simulink model "MSIP_Speed_Control_abc1a_2025a_no_VSC_no_Bspline"  (R2025a)
settings: Solver=FixedStepAuto  StartTime=0.0  StopTime=150  FixedStep=1e-4  MaxStep=1e-3  RelTol=1e-3
model workspace (MAT data in the model file):
  Freq = 60
values from neighbouring files (symbols this model uses):
  alpha0_wMS = (b_MS*Rs_MS/(J_MS*Lq_MS)) +               (3*np_MS*np_MS*lambda_MS*lambda_MS/              (2*J_MS*Lq_MS))    (= 296.519413831)    [data_MSIP_julio2025.m]
  alpha1_wMS = (Rs_MS/Lq_MS) + (b_MS/J_MS)    (= 7.15599341383)    [data_MSIP_julio2025.m]
  b_MS = 1e-3    (= 0.001)    [data_MSIP_julio2025.m]
  beta0_wMS = Pw^2    (= 400)    [data_MSIP_julio2025.m]
  beta1_wMS = 2*Pw    (= 40)    [data_MSIP_julio2025.m]
  beta_d_MS = pd_MS    (= 40)    [data_MSIP_julio2025.m]
  gamq = 2*J_MS*Lq_MS/(3*np_MS*lambda_MS)    (= 0.00452625826005)    [data_MSIP_julio2025.m]
  J_MS = 1e-1    (= 0.1)    [data_MSIP_julio2025.m]
  lambda_MS = 67.09e-2    (= 0.6709)    [data_MSIP_julio2025.m]
  Ld_MS = 22.1e-3    (= 0.0221)    [data_MSIP_julio2025.m]
  Lq_MS = 91.1e-3    (= 0.0911)    [data_MSIP_julio2025.m]
  np_MS = 2    [data_MSIP_julio2025.m]
  Rs_MS = 6.51e-1    (= 0.651)    [data_MSIP_julio2025.m]
undefined symbols (not defined in the file or in its folder): plecs
libraries: plecslib_extras2 x2, spsRMSLib x2
settings Model: SimulationMode=accelerator  PauseTimes=0.01  Creator=RUBEN TAPIA OLVERA  LastModifiedBy=avalder
settings SolverCC: AlgebraicLoopSolver=TrustRegion
settings DataIOCC: ReturnWorkspaceOutputs=off
settings OptimizationCC: LifeSpan=inf
settings DebuggingCC: MaxConsecutiveZCsMsg=none  UnconnectedInputMsg=warning  UnconnectedOutputMsg=warning  UnconnectedLineMsg=warning  SFUnexpectedBacktrackingDiag=warning  SFNoUnconditionalDefaultTransitionDiag=warning  SFExecutionAtInitializationDiag=none  ArithmeticOperatorsInVariantConditions=warning
settings ModelReferenceCC: EnableRefExpFcnMdlSchedulingChecks=on
settings SFSimCC: SimUseLocalCustomCode=off  CustomCodeUndefinedFunction=UseInterfaceOnly
settings RTWCC: RTWUseLocalCustomCode=off  GPUComputeCapability=3.5
settings CodeAppCC: StateflowObjectComments=on
settings GRTTargetCC: TargetLangStandard=C89/C90 (ANSI)
settings ConfigComp: CovMetricSettings=dw  CovSaveCumulativeToWorkspaceVar=on  CovSaveSingleToWorkspaceVar=on  CovExternalEMLEnable=off
settings SimscapeCC: SimscapeNormalizeSystem=off

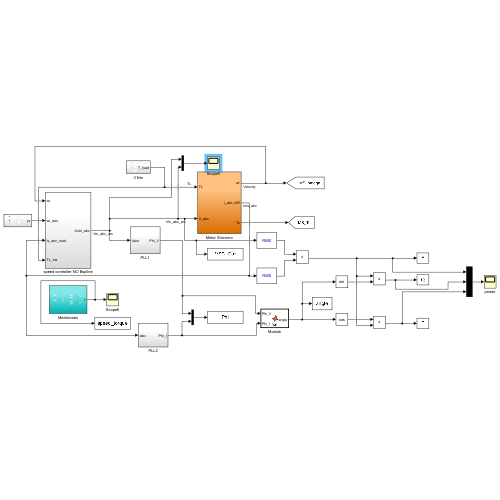
[thumbnail: Simulink's stored preview of the top-level diagram]
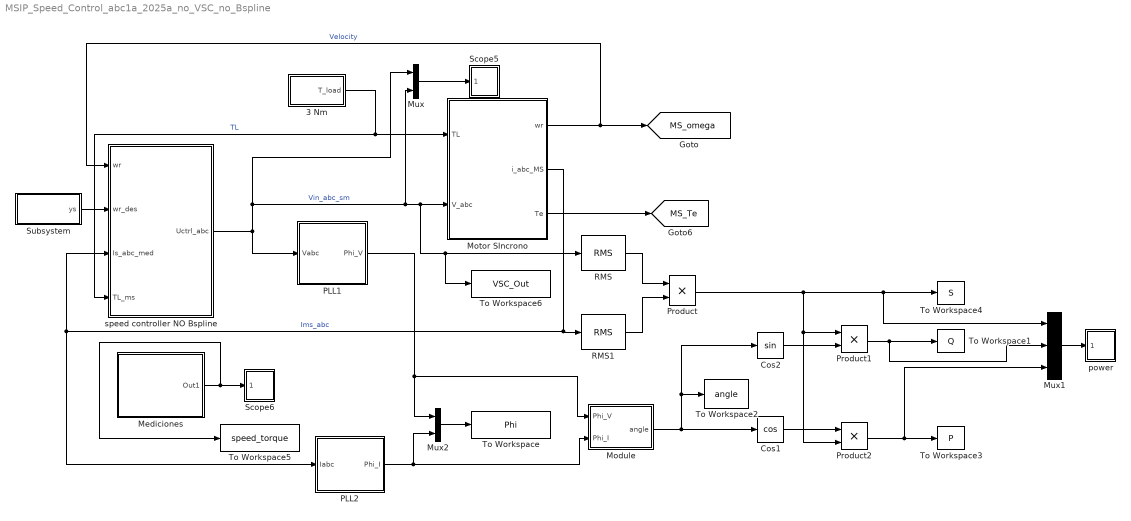
== system MSIP_Speed_Control_abc1a_2025a_no_VSC_no_Bspline ==
  3 Nm : Subsystem
  Cos1 : Trigonometry  Operator=cos
  Cos2 : Trigonometry
  Mediciones : Subsystem
  Module : MATLAB Function  TreatAsAtomicUnit=on
  Motor SIncrono : Subsystem
  Mux : Mux  Inputs=2
  Mux1 : Mux  Inputs=3
  Mux2 : Mux  Inputs=2
  PLL1 : Subsystem
  PLL2 : Subsystem
  Product : Product
  Product1 : Product
  Product2 : Product
  RMS : spsRMSLib/RMS  TrueRMS=on  Freq=Freq  RMSInit=0  Ts=0
  RMS1 : spsRMSLib/RMS  TrueRMS=on  Freq=Freq  RMSInit=0  Ts=0
  Scope5 : Subsystem  LoadFcn=plecs('sl', 300);  InitFcn=plecs('sl', 314);  StartFcn=plecs('sl', 308);  StopFcn=plecs('sl', 309);  mask{Settings=<binary blob, 776 chars, not shown>}
      mask init:
      | plecs('sl', 315);
      settings: CopyFcn=plecs('sl', 303);  DeleteFcn=plecs('sl', 305);  UndoDeleteFcn=plecs('sl', 306);  PreSaveFcn=plecs('sl', 311);  NameChangeFcn=plecs('sl', 310);  DestroyFcn=plecs('sl', 307);  OpenFcn=plecs('sl', 302);  ErrorFcn=plerrorfcn
      mask Display: plot([0.1 0.9 0.9 0.1 0.1], [0.9 0.9 0.5 0.5 0.9])
  Scope6 : Subsystem  LoadFcn=plecs('sl', 300);  InitFcn=plecs('sl', 314);  StartFcn=plecs('sl', 308);  StopFcn=plecs('sl', 309);  mask{Settings=<binary blob, 752 chars, not shown>}
      mask init:
      | plecs('sl', 315);
      settings: CopyFcn=plecs('sl', 303);  DeleteFcn=plecs('sl', 305);  UndoDeleteFcn=plecs('sl', 306);  PreSaveFcn=plecs('sl', 311);  NameChangeFcn=plecs('sl', 310);  DestroyFcn=plecs('sl', 307);  OpenFcn=plecs('sl', 302);  ErrorFcn=plerrorfcn
      mask Display: plot([0.1 0.9 0.9 0.1 0.1], [0.9 0.9 0.5 0.5 0.9])
  Subsystem : Subsystem
  To Workspace : ToWorkspace  VariableName=Phi  SaveFormat=Timeseries  SampleTime=-1
  To Workspace1 : ToWorkspace  VariableName=Q  SaveFormat=Timeseries  SampleTime=-1
  To Workspace2 : ToWorkspace  VariableName=angle  SaveFormat=Timeseries  SampleTime=-1
  To Workspace3 : ToWorkspace  VariableName=P  SaveFormat=Timeseries  SampleTime=-1
  To Workspace4 : ToWorkspace  VariableName=S  SaveFormat=Timeseries  SampleTime=-1
  To Workspace5 : ToWorkspace  VariableName=speed_torque  SaveFormat=Timeseries  SampleTime=-1
  To Workspace6 : ToWorkspace  VariableName=VSC_Out  SaveFormat=Timeseries  SampleTime=-1
  power : Subsystem  LoadFcn=plecs('sl', 300);  InitFcn=plecs('sl', 314);  StartFcn=plecs('sl', 308);  StopFcn=plecs('sl', 309);  mask{Settings=<binary blob, 756 chars, not shown>}
      mask init:
      | plecs('sl', 315);
      settings: CopyFcn=plecs('sl', 303);  DeleteFcn=plecs('sl', 305);  UndoDeleteFcn=plecs('sl', 306);  PreSaveFcn=plecs('sl', 311);  NameChangeFcn=plecs('sl', 310);  DestroyFcn=plecs('sl', 307);  OpenFcn=plecs('sl', 302);  ErrorFcn=plerrorfcn
      mask Display: plot([0.1 0.9 0.9 0.1 0.1], [0.9 0.9 0.5 0.5 0.9])
  speed controller NO Bspline : Subsystem
  tag scope: MS_Te=global, MS_omega=global
  wires:
  Motor SIncrono/1(wr) -> speed controller NO Bspline/1(wr), [MS_omega]  "Velocity"
  3 Nm/1(T_load) -> speed controller NO Bspline/4(TL_ms), Motor SIncrono/1(TL)  "TL"
  Motor SIncrono/3(Te) -> [MS_Te]
  Motor SIncrono/2(i_abc_MS) -> RMS1/1, speed controller NO Bspline/3(Is_abc_med), PLL2/1(Iabc)  "Ims_abc"
  Subsystem/1(ys) -> speed controller NO Bspline/2(wr_des)
  Mux2/1 -> To Workspace/1
  Module/1(angle) -> Cos1/1, To Workspace2/1, Cos2/1
  PLL1/1(Phi_V) -> Mux2/1, Module/1(Phi_V)
  PLL2/1(Phi_I) -> Module/2(Phi_I), Mux2/2
  speed controller NO Bspline/1(Uctrl_abc) -> Mux/2, Motor SIncrono/2(V_abc), To Workspace6/1, RMS/1, Mux/1, PLL1/1(Vabc)  "Vin_abc_sm"
  Product/1 -> Product2/2, Product1/1, Mux1/1, To Workspace4/1
  RMS/1 -> Product/1
  RMS1/1 -> Product/2
  Mux/1 -> Scope5/1(1)
  Mediciones/1(Out1) -> To Workspace5/1, Scope6/1(1)
  Cos2/1 -> Product1/2
  Cos1/1 -> Product2/1
  Product1/1 -> Mux1/2, To Workspace1/1
  Product2/1 -> Mux1/3, To Workspace3/1
  Mux1/1 -> power/1(1)

== system MSIP_Speed_Control_abc1a_2025a_no_VSC_no_Bspline/3 Nm ==
  Add : Sum  Inputs=+++
  TL1 : MATLAB Function  TreatAsAtomicUnit=on
  TL2 : MATLAB Function  TreatAsAtomicUnit=on
  TL3 : MATLAB Function  TreatAsAtomicUnit=on
  Tiempo1 : Clock
  T_load : Outport
  tag scope: TL_MS=global
  wires:
  Tiempo1/1 -> TL3/1(t), TL2/1(t), TL1/1(t)
  TL3/1(T_load3) -> Add/3
  TL1/1(T_load) -> Add/1
  TL2/1(T_load2) -> Add/2
  Add/1 -> T_load/1, [TL_MS]

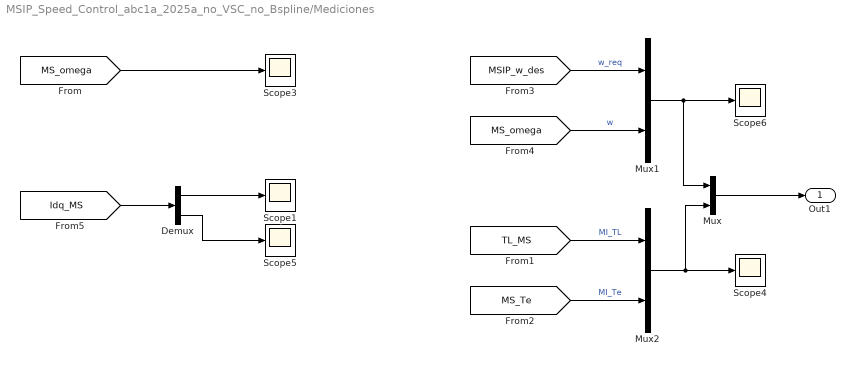
== system MSIP_Speed_Control_abc1a_2025a_no_VSC_no_Bspline/Mediciones ==
  Demux : Demux  Outputs=2
  Mux : Mux  Inputs=2
  Mux1 : Mux  Inputs=2
  Mux2 : Mux  Inputs=2
  Scope{1,3..6} (5 alike) : Scope
      Scope1 settings: Title=Currents  ActiveDisplayYMinimum=-0.00105  ActiveDisplayYMaximum=0.01123  DataLoggingVariableName=ScopeData3
      Scope3 settings: ActiveDisplayYMinimum=-1  ActiveDisplayYMaximum=1
      Scope4 settings: ActiveDisplayYMinimum=-1  ActiveDisplayYMaximum=1  DataLoggingVariableName=ScopeData4
      Scope5 settings: Title=Currents  ActiveDisplayYMinimum=-0.003  ActiveDisplayYMaximum=0.00033
      Scope6 settings: ActiveDisplayYMinimum=-23.57031  ActiveDisplayYMaximum=212.1328
  Out1 : Outport
  wires:
  [MS_omega] -> Scope3/1
  [TL_MS] -> Mux2/1  "MI_TL"
  Mux2/1 -> Mux/2, Scope4/1
  [MS_Te] -> Mux2/2  "MI_Te"
  [Idq_MS] -> Demux/1
  Demux/1 -> Scope1/1
  Demux/2 -> Scope5/1
  [MS_omega] -> Mux1/2  "w"
  [MSIP_w_des] -> Mux1/1  "w_req"
  Mux1/1 -> Mux/1, Scope6/1
  Mux/1 -> Out1/1

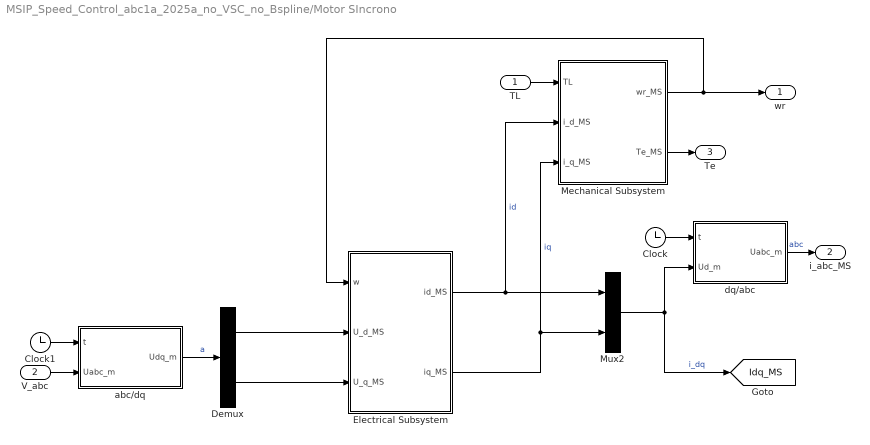
== system MSIP_Speed_Control_abc1a_2025a_no_VSC_no_Bspline/Motor SIncrono ==
  TL : Inport
  V_abc : Inport  Port=2
  Clock : Clock
  Clock1 : Clock
  Demux : Demux  Outputs=2
  Electrical Subsystem : Subsystem
  Mechanical Subsystem : Subsystem
  Mux2 : Mux  Inputs=2
  abc/dq : Subsystem
  dq/abc : Subsystem
  wr : Outport
  i_abc_MS : Outport  Port=2
  Te : Outport  Port=3
  tag scope: Idq_MS=global
  wires:
  Mechanical Subsystem/1(wr_MS) -> wr/1, Electrical Subsystem/1(w)
  TL/1 -> Mechanical Subsystem/1(TL)
  Mechanical Subsystem/2(Te_MS) -> Te/1
  Demux/1 -> Electrical Subsystem/2(U_d_MS)
  Demux/2 -> Electrical Subsystem/3(U_q_MS)
  Electrical Subsystem/1(id_MS) -> Mux2/1, Mechanical Subsystem/2(i_d_MS)  "id"
  Electrical Subsystem/2(iq_MS) -> Mechanical Subsystem/3(i_q_MS), Mux2/2  "iq"
  Mux2/1 -> dq/abc/2(Ud_m), [Idq_MS]  "i_dq"
  Clock/1 -> dq/abc/1(t)
  dq/abc/1(Uabc_m) -> i_abc_MS/1  "abc"
  Clock1/1 -> abc/dq/1(t)
  abc/dq/1(Udq_m) -> Demux/1  "a"
  V_abc/1 -> abc/dq/2(Uabc_m)

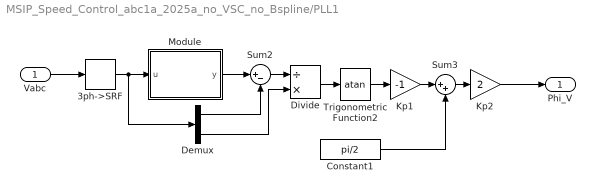
== system MSIP_Speed_Control_abc1a_2025a_no_VSC_no_Bspline/PLL1 ==
  Vabc : Inport
  3ph->SRF : plecslib_extras2/Transformations/3ph->SRF
      settings: SourceProductName=PLECS Extras
  Constant1 : Constant  Value=pi/2
  Demux : Demux  Outputs=2
  Divide : Product  Inputs=/*
  Kp1 : Gain  Gain=-1  SaturateOnIntegerOverflow=on  OutDataTypeStr=Inherit: Same as input  ParamDataTypeStr=Inherit: Same as input
  Kp2 : Gain  Gain=2  SaturateOnIntegerOverflow=on  OutDataTypeStr=Inherit: Same as input  ParamDataTypeStr=Inherit: Same as input
  Module : MATLAB Function  TreatAsAtomicUnit=on
  Sum2 : Sum  Inputs=|+-
  Sum3 : Sum  Inputs=|++
  Trigonometric Function2 : Trigonometry  Operator=atan
  Phi_V : Outport
  wires:
  Demux/2 -> Divide/2
  Vabc/1 -> 3ph->SRF/1
  Demux/1 -> Sum2/2
  Sum2/1 -> Divide/1
  Divide/1 -> Trigonometric Function2/1
  Sum3/1 -> Kp2/1
  Module/1(y) -> Sum2/1
  Kp2/1 -> Phi_V/1
  Trigonometric Function2/1 -> Kp1/1
  Kp1/1 -> Sum3/1
  Constant1/1 -> Sum3/2
  3ph->SRF/1 -> Demux/1, Module/1(u)

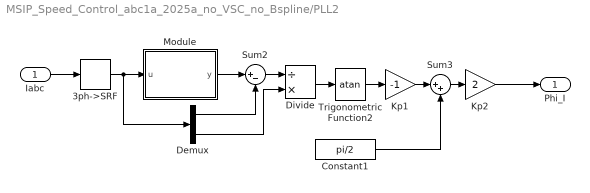
== system MSIP_Speed_Control_abc1a_2025a_no_VSC_no_Bspline/PLL2 ==
  Iabc : Inport
  3ph->SRF : plecslib_extras2/Transformations/3ph->SRF
      settings: SourceProductName=PLECS Extras
  Constant1 : Constant  Value=pi/2
  Demux : Demux  Outputs=2
  Divide : Product  Inputs=/*
  Kp1 : Gain  Gain=-1  SaturateOnIntegerOverflow=on  OutDataTypeStr=Inherit: Same as input  ParamDataTypeStr=Inherit: Same as input
  Kp2 : Gain  Gain=2  SaturateOnIntegerOverflow=on  OutDataTypeStr=Inherit: Same as input  ParamDataTypeStr=Inherit: Same as input
  Module : MATLAB Function  TreatAsAtomicUnit=on
  Sum2 : Sum  Inputs=|+-
  Sum3 : Sum  Inputs=|++
  Trigonometric Function2 : Trigonometry  Operator=atan
  Phi_I : Outport
  wires:
  Demux/2 -> Divide/2
  Iabc/1 -> 3ph->SRF/1
  Demux/1 -> Sum2/2
  Sum2/1 -> Divide/1
  Divide/1 -> Trigonometric Function2/1
  Sum3/1 -> Kp2/1
  Module/1(y) -> Sum2/1
  Kp2/1 -> Phi_I/1
  Trigonometric Function2/1 -> Kp1/1
  Kp1/1 -> Sum3/1
  Constant1/1 -> Sum3/2
  3ph->SRF/1 -> Demux/1, Module/1(u)

== system MSIP_Speed_Control_abc1a_2025a_no_VSC_no_Bspline/Scope5 ==
  1 : Inport
  " InputMux " : Subsystem
      mask Display: disp('Mux')
  " S-Function " : S-Function  FunctionName=plecs  SFunctionDeploymentMode=off  EnableBusSupport=off
  wires:
  1/1 -> " InputMux "/1(In1)
  " InputMux "/1(Out) -> " S-Function "/1

== system MSIP_Speed_Control_abc1a_2025a_no_VSC_no_Bspline/Scope6 ==
  1 : Inport
  " InputMux " : Subsystem
      mask Display: disp('Mux')
  " S-Function " : S-Function  FunctionName=plecs  SFunctionDeploymentMode=off  EnableBusSupport=off
  wires:
  1/1 -> " InputMux "/1(In1)
  " InputMux "/1(Out) -> " S-Function "/1

== system MSIP_Speed_Control_abc1a_2025a_no_VSC_no_Bspline/Subsystem ==
  Add : Sum  Inputs=+++
  Theta_Deseada : MATLAB Function  TreatAsAtomicUnit=on
  Theta_Deseada1 : MATLAB Function  TreatAsAtomicUnit=on
  Theta_Deseada2 : MATLAB Function  TreatAsAtomicUnit=on
  Tiempo1 : Clock
  ys : Outport
  tag scope: MSIP_w_des=global
  wires:
  Tiempo1/1 -> Theta_Deseada1/1(t), Theta_Deseada2/1(t), Theta_Deseada/1(t)
  Theta_Deseada/1(ys) -> Add/1
  Theta_Deseada1/1(ys) -> Add/2
  Theta_Deseada2/1(ys) -> Add/3
  Add/1 -> ys/1, [MSIP_w_des]

== system MSIP_Speed_Control_abc1a_2025a_no_VSC_no_Bspline/power ==
  1 : Inport
  " InputMux " : Subsystem
      mask Display: disp('Mux')
  " S-Function " : S-Function  FunctionName=plecs  SFunctionDeploymentMode=off  EnableBusSupport=off
  wires:
  1/1 -> " InputMux "/1(In1)
  " InputMux "/1(Out) -> " S-Function "/1

== system MSIP_Speed_Control_abc1a_2025a_no_VSC_no_Bspline/speed controller NO Bspline ==
  wr : Inport
  wr_des : Inport  Port=2
  Is_abc_med : Inport  Port=3
  TL_ms : Inport  Port=4
  Clock : Clock
  Mux : Mux  Inputs=2
  control loop U_wr : Subsystem
  dq/abc : Subsystem
  Uctrl_abc : Outport
  tag scope: Vin_MS=global
  wires:
  wr/1 -> control loop U_wr/2(wr)
  wr_des/1 -> control loop U_wr/1(wr_ref)
  TL_ms/1 -> control loop U_wr/4(TLms)
  Is_abc_med/1 -> control loop U_wr/3(Ims_abc)
  control loop U_wr/1(U1_d) -> Mux/1  "U_theta"
  control loop U_wr/2(U1_q) -> Mux/2
  Clock/1 -> dq/abc/1(t)
  Mux/1 -> dq/abc/2(Ud_m), [Vin_MS]  "i_dq"
  dq/abc/1(Uabc_m) -> Uctrl_abc/1  "abc"

== system MSIP_Speed_Control_abc1a_2025a_no_VSC_no_Bspline/Motor SIncrono/Electrical Subsystem ==
  w : Inport
  U_d_MS : Inport  Port=2
  U_q_MS : Inport  Port=3
  Currents : Subsystem
  id_MS : Outport
  iq_MS : Outport  Port=2
  wires:
  w/1 -> Currents/1(w)
  Currents/1(id_Msinc) -> id_MS/1
  Currents/2(iq_Msinc) -> iq_MS/1
  U_d_MS/1 -> Currents/2(UdMS)
  U_q_MS/1 -> Currents/3(UqMS)

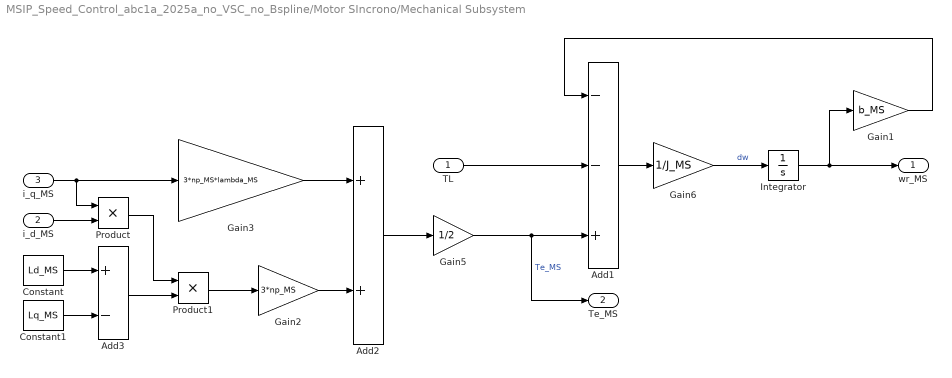
== system MSIP_Speed_Control_abc1a_2025a_no_VSC_no_Bspline/Motor SIncrono/Mechanical Subsystem ==
  TL : Inport
  i_d_MS : Inport  Port=2
  i_q_MS : Inport  Port=3
  Add1 : Sum  Inputs=--+
  Add2 : Sum
  Add3 : Sum  Inputs=+-
  Constant : Constant  Value=Ld_MS
  Constant1 : Constant  Value=Lq_MS
  Gain1 : Gain  Gain=b_MS
  Gain2 : Gain  Gain=3*np_MS
  Gain3 : Gain  Gain=3*np_MS*lambda_MS
  Gain5 : Gain  Gain=1/2
  Gain6 : Gain  Gain=1/J_MS
  Integrator : Integrator
  Product : Product
  Product1 : Product
  wr_MS : Outport
  Te_MS : Outport  Port=2
  wires:
  Gain5/1 -> Te_MS/1, Add1/3  "Te_MS"
  Gain2/1 -> Add2/2
  TL/1 -> Add1/2
  i_d_MS/1 -> Product/2
  Product1/1 -> Gain2/1
  Gain3/1 -> Add2/1
  Gain1/1 -> Add1/1
  Add3/1 -> Product1/2
  Product/1 -> Product1/1
  Constant1/1 -> Add3/2
  Constant/1 -> Add3/1
  i_q_MS/1 -> Product/1, Gain3/1
  Add2/1 -> Gain5/1
  Integrator/1 -> wr_MS/1, Gain1/1
  Add1/1 -> Gain6/1
  Gain6/1 -> Integrator/1  "dw"

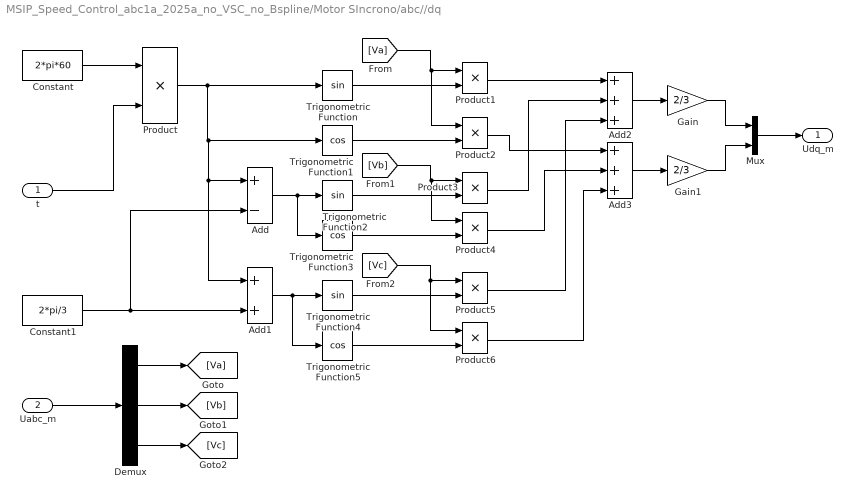
== system MSIP_Speed_Control_abc1a_2025a_no_VSC_no_Bspline/Motor SIncrono/abc//dq ==
  t : Inport
  Uabc_m : Inport  Port=2
  Add : Sum  Inputs=+-
  Add1 : Sum
  Add2 : Sum  Inputs=+++
  Add3 : Sum  Inputs=+++
  Constant : Constant  Value=2*pi*60
  Constant1 : Constant  Value=2*pi/3
  Demux : Demux  Outputs=3
  Gain : Gain  Gain=2/3
  Gain1 : Gain  Gain=2/3
  Mux : Mux  Inputs=2
  Product{,1..6} (7 alike) : Product
  Trigonometric Function : Trigonometry
  Trigonometric Function1 : Trigonometry  Operator=cos
  Trigonometric Function2 : Trigonometry
  Trigonometric Function3 : Trigonometry  Operator=cos
  Trigonometric Function4 : Trigonometry
  Trigonometric Function5 : Trigonometry  Operator=cos
  Udq_m : Outport
  wires:
  t/1 -> Product/2
  Constant/1 -> Product/1
  Product/1 -> Add1/1, Add/1, Trigonometric Function1/1, Trigonometric Function/1
  Constant1/1 -> Add1/2, Add/2
  Add/1 -> Trigonometric Function3/1, Trigonometric Function2/1
  Add1/1 -> Trigonometric Function5/1, Trigonometric Function4/1
  Trigonometric Function/1 -> Product1/2
  Trigonometric Function2/1 -> Product3/2
  Uabc_m/1 -> Demux/1
  Add2/1 -> Gain/1
  Add3/1 -> Gain1/1
  Demux/1 -> [Va]
  Demux/2 -> [Vb]
  Demux/3 -> [Vc]
  [Va] -> Product2/1, Product1/1
  Product1/1 -> Add2/1
  [Vb] -> Product4/1, Product3/1
  Product3/1 -> Add2/2
  Trigonometric Function4/1 -> Product5/2
  [Vc] -> Product6/1, Product5/1
  Product5/1 -> Add2/3
  Product2/1 -> Add3/1
  Trigonometric Function5/1 -> Product6/2
  Trigonometric Function3/1 -> Product4/2
  Trigonometric Function1/1 -> Product2/2
  Product4/1 -> Add3/2
  Product6/1 -> Add3/3
  Mux/1 -> Udq_m/1
  Gain/1 -> Mux/1
  Gain1/1 -> Mux/2

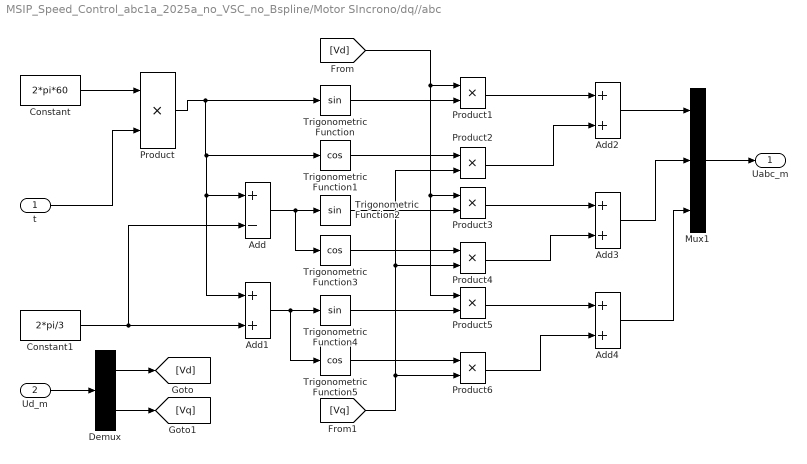
== system MSIP_Speed_Control_abc1a_2025a_no_VSC_no_Bspline/Motor SIncrono/dq//abc ==
  t : Inport
  Ud_m : Inport  Port=2
  Add : Sum  Inputs=+-
  Add{1..4} (4 alike) : Sum
  Constant : Constant  Value=2*pi*60
  Constant1 : Constant  Value=2*pi/3
  Demux : Demux  Outputs=2
  Mux1 : Mux  Inputs=3
  Product{,1..6} (7 alike) : Product
  Trigonometric Function : Trigonometry
  Trigonometric Function1 : Trigonometry  Operator=cos
  Trigonometric Function2 : Trigonometry
  Trigonometric Function3 : Trigonometry  Operator=cos
  Trigonometric Function4 : Trigonometry
  Trigonometric Function5 : Trigonometry  Operator=cos
  Uabc_m : Outport
  wires:
  t/1 -> Product/2
  Constant/1 -> Product/1
  Product/1 -> Add1/1, Add/1, Trigonometric Function1/1, Trigonometric Function/1
  Constant1/1 -> Add1/2, Add/2
  Add/1 -> Trigonometric Function3/1, Trigonometric Function2/1
  Add1/1 -> Trigonometric Function5/1, Trigonometric Function4/1
  Trigonometric Function/1 -> Product1/2
  Trigonometric Function1/1 -> Product2/1
  Product1/1 -> Add2/1
  Product2/1 -> Add2/2
  Trigonometric Function2/1 -> Product3/2
  Trigonometric Function3/1 -> Product4/1
  Product3/1 -> Add3/1
  Product4/1 -> Add3/2
  Trigonometric Function4/1 -> Product5/2
  Trigonometric Function5/1 -> Product6/1
  Product5/1 -> Add4/1
  Product6/1 -> Add4/2
  Mux1/1 -> Uabc_m/1
  Add2/1 -> Mux1/1
  Add3/1 -> Mux1/2
  Add4/1 -> Mux1/3
  Ud_m/1 -> Demux/1
  Demux/1 -> [Vd]
  Demux/2 -> [Vq]
  [Vd] -> Product5/1, Product3/1, Product1/1
  [Vq] -> Product4/2, Product2/2, Product6/2

== system MSIP_Speed_Control_abc1a_2025a_no_VSC_no_Bspline/Scope5/ InputMux  ==
  In1 : Inport
  Convert1 : DataTypeConversion
  Mux : Mux  Inputs=1
  Out : Outport
  wires:
  Convert1/1 -> Mux/1
  In1/1 -> Convert1/1
  Mux/1 -> Out/1

== system MSIP_Speed_Control_abc1a_2025a_no_VSC_no_Bspline/Scope6/ InputMux  ==
  In1 : Inport
  Convert1 : DataTypeConversion
  Mux : Mux  Inputs=1
  Out : Outport
  wires:
  Convert1/1 -> Mux/1
  In1/1 -> Convert1/1
  Mux/1 -> Out/1

== system MSIP_Speed_Control_abc1a_2025a_no_VSC_no_Bspline/power/ InputMux  ==
  In1 : Inport
  Convert1 : DataTypeConversion
  Mux : Mux  Inputs=1
  Out : Outport
  wires:
  Convert1/1 -> Mux/1
  In1/1 -> Convert1/1
  Mux/1 -> Out/1

== system MSIP_Speed_Control_abc1a_2025a_no_VSC_no_Bspline/speed controller NO Bspline/control loop U_wr ==
  wr_ref : Inport
  wr : Inport  Port=2
  Ims_abc : Inport  Port=3
  TLms : Inport  Port=4
  Clock : Clock
  Ctrl unit U1_d : Subsystem
  Ctrl unit U1_d1 : Subsystem
  abc/dq : Subsystem
  U1_d : Outport
  U1_q : Outport  Port=2
  wires:
  wr/1 -> Ctrl unit U1_d1/2(wr), Ctrl unit U1_d/1(wr)
  TLms/1 -> Ctrl unit U1_d1/3(MS_TL)
  Ims_abc/1 -> abc/dq/2(Uabc_m)
  Clock/1 -> abc/dq/1(t)
  abc/dq/1(Udq_m) -> Ctrl unit U1_d/2(MS_Idq)  "a"
  Ctrl unit U1_d/1(ud) -> U1_d/1
  Ctrl unit U1_d1/1(uq) -> U1_q/1
  wr_ref/1 -> Ctrl unit U1_d1/1(MSwr_des)

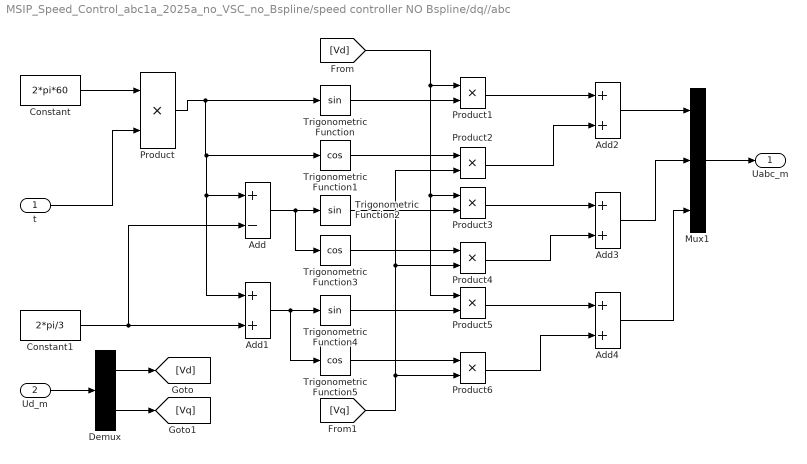
== system MSIP_Speed_Control_abc1a_2025a_no_VSC_no_Bspline/speed controller NO Bspline/dq//abc ==
  t : Inport
  Ud_m : Inport  Port=2
  Add : Sum  Inputs=+-
  Add{1..4} (4 alike) : Sum
  Constant : Constant  Value=2*pi*60
  Constant1 : Constant  Value=2*pi/3
  Demux : Demux  Outputs=2
  Mux1 : Mux  Inputs=3
  Product{,1..6} (7 alike) : Product
  Trigonometric Function : Trigonometry
  Trigonometric Function1 : Trigonometry  Operator=cos
  Trigonometric Function2 : Trigonometry
  Trigonometric Function3 : Trigonometry  Operator=cos
  Trigonometric Function4 : Trigonometry
  Trigonometric Function5 : Trigonometry  Operator=cos
  Uabc_m : Outport
  wires:
  t/1 -> Product/2
  Constant/1 -> Product/1
  Product/1 -> Add1/1, Add/1, Trigonometric Function1/1, Trigonometric Function/1
  Constant1/1 -> Add1/2, Add/2
  Add/1 -> Trigonometric Function3/1, Trigonometric Function2/1
  Add1/1 -> Trigonometric Function5/1, Trigonometric Function4/1
  Trigonometric Function/1 -> Product1/2
  Trigonometric Function1/1 -> Product2/1
  Product1/1 -> Add2/1
  Product2/1 -> Add2/2
  Trigonometric Function2/1 -> Product3/2
  Trigonometric Function3/1 -> Product4/1
  Product3/1 -> Add3/1
  Product4/1 -> Add3/2
  Trigonometric Function4/1 -> Product5/2
  Trigonometric Function5/1 -> Product6/1
  Product5/1 -> Add4/1
  Product6/1 -> Add4/2
  Mux1/1 -> Uabc_m/1
  Add2/1 -> Mux1/1
  Add3/1 -> Mux1/2
  Add4/1 -> Mux1/3
  Ud_m/1 -> Demux/1
  Demux/1 -> [Vd]
  Demux/2 -> [Vq]
  [Vd] -> Product5/1, Product3/1, Product1/1
  [Vq] -> Product4/2, Product2/2, Product6/2

== system MSIP_Speed_Control_abc1a_2025a_no_VSC_no_Bspline/Motor SIncrono/Electrical Subsystem/Currents ==
  w : Inport
  UdMS : Inport  Port=2
  UqMS : Inport  Port=3
  Subsystem : Subsystem
  Subsystem1 : Subsystem
  id_Msinc : Outport
  iq_Msinc : Outport  Port=2
  wires:
  w/1 -> Subsystem1/1(wrMS), Subsystem/1(wrMS)
  UdMS/1 -> Subsystem/2(udMS)
  Subsystem/1(idMS) -> Subsystem1/3(idMS), id_Msinc/1
  Subsystem1/1(iq_Msinc) -> Subsystem/3(iqMS), iq_Msinc/1
  UqMS/1 -> Subsystem1/2(uqMS)

== system MSIP_Speed_Control_abc1a_2025a_no_VSC_no_Bspline/speed controller NO Bspline/control loop U_wr/Ctrl unit U1_d ==
  wr : Inport
  MS_Idq : Inport  Port=2
  Add1 : Sum  Inputs=--
  Demux : Demux  Outputs=2
  Gain1 : Gain  Gain=beta_d_MS
  Gain2 : Gain  Gain=Lq_MS*np_MS
  Product : Product
  ud : Outport
  wires:
  Add1/1 -> ud/1
  MS_Idq/1 -> Demux/1
  Demux/1 -> Gain1/1  "Id"
  Demux/2 -> Product/2  "Iq"
  Gain1/1 -> Add1/1
  wr/1 -> Product/1
  Product/1 -> Gain2/1
  Gain2/1 -> Add1/2

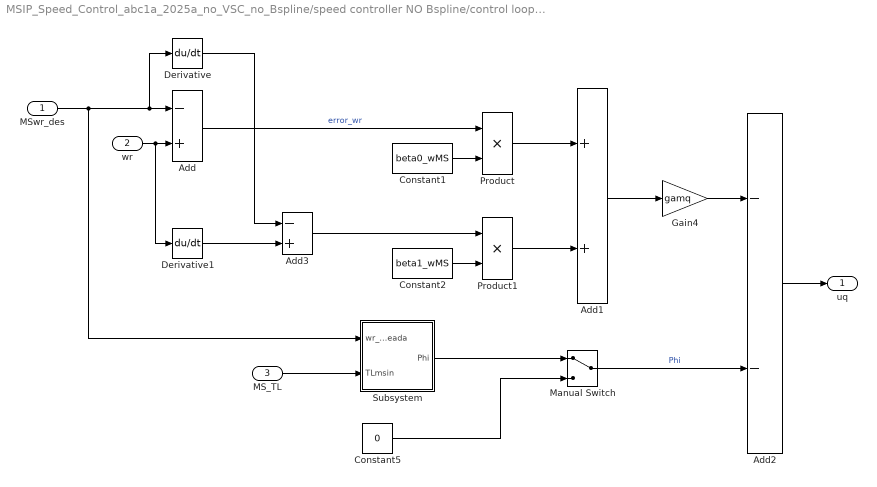
== system MSIP_Speed_Control_abc1a_2025a_no_VSC_no_Bspline/speed controller NO Bspline/control loop U_wr/Ctrl unit U1_d1 ==
  MSwr_des : Inport
  wr : Inport  Port=2
  MS_TL : Inport  Port=3
  Add : Sum  Inputs=-+
  Add1 : Sum
  Add2 : Sum  Inputs=--
  Add3 : Sum  Inputs=-+
  Constant1 : Constant  Value=beta0_wMS
  Constant2 : Constant  Value=beta1_wMS
  Constant5 : Constant  Value=0
  Derivative : Derivative
  Derivative1 : Derivative
  Gain4 : Gain  Gain=gamq
  Manual Switch : ManualSwitch
  Product : Product
  Product1 : Product
  Subsystem : Subsystem
  uq : Outport
  wires:
  MSwr_des/1 -> Subsystem/1(wr_deseada), Derivative/1, Add/1
  wr/1 -> Derivative1/1, Add/2
  Constant5/1 -> Manual Switch/2
  Manual Switch/1 -> Add2/2  "Phi"
  Add/1 -> Product/1  "error_wr"
  Product1/1 -> Add1/2
  Product/1 -> Add1/1
  MS_TL/1 -> Subsystem/2(TLmsin)
  Constant1/1 -> Product/2
  Add3/1 -> Product1/1
  Derivative/1 -> Add3/1
  Constant2/1 -> Product1/2
  Add2/1 -> uq/1
  Add1/1 -> Gain4/1
  Gain4/1 -> Add2/1
  Derivative1/1 -> Add3/2
  Subsystem/1(Phi) -> Manual Switch/1

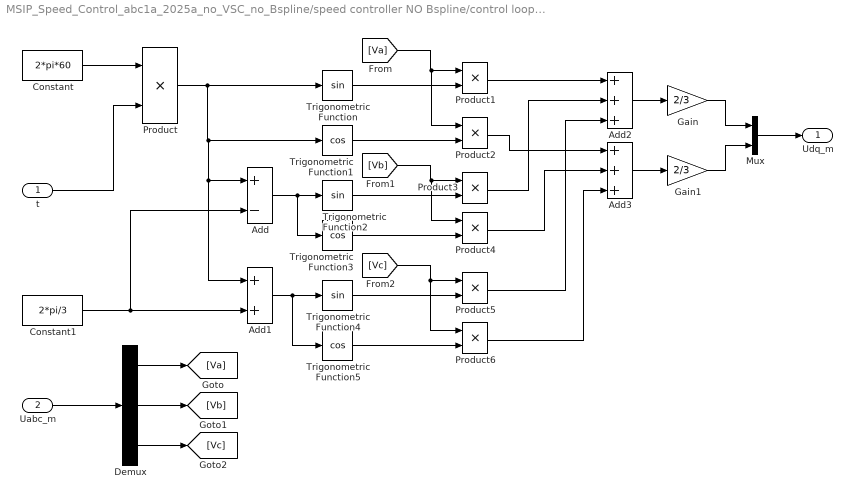
== system MSIP_Speed_Control_abc1a_2025a_no_VSC_no_Bspline/speed controller NO Bspline/control loop U_wr/abc//dq ==
  t : Inport
  Uabc_m : Inport  Port=2
  Add : Sum  Inputs=+-
  Add1 : Sum
  Add2 : Sum  Inputs=+++
  Add3 : Sum  Inputs=+++
  Constant : Constant  Value=2*pi*60
  Constant1 : Constant  Value=2*pi/3
  Demux : Demux  Outputs=3
  Gain : Gain  Gain=2/3
  Gain1 : Gain  Gain=2/3
  Mux : Mux  Inputs=2
  Product{,1..6} (7 alike) : Product
  Trigonometric Function : Trigonometry
  Trigonometric Function1 : Trigonometry  Operator=cos
  Trigonometric Function2 : Trigonometry
  Trigonometric Function3 : Trigonometry  Operator=cos
  Trigonometric Function4 : Trigonometry
  Trigonometric Function5 : Trigonometry  Operator=cos
  Udq_m : Outport
  wires:
  t/1 -> Product/2
  Constant/1 -> Product/1
  Product/1 -> Add1/1, Add/1, Trigonometric Function1/1, Trigonometric Function/1
  Constant1/1 -> Add1/2, Add/2
  Add/1 -> Trigonometric Function3/1, Trigonometric Function2/1
  Add1/1 -> Trigonometric Function5/1, Trigonometric Function4/1
  Trigonometric Function/1 -> Product1/2
  Trigonometric Function2/1 -> Product3/2
  Uabc_m/1 -> Demux/1
  Add2/1 -> Gain/1
  Add3/1 -> Gain1/1
  Demux/1 -> [Va]
  Demux/2 -> [Vb]
  Demux/3 -> [Vc]
  [Va] -> Product2/1, Product1/1
  Product1/1 -> Add2/1
  [Vb] -> Product4/1, Product3/1
  Product3/1 -> Add2/2
  Trigonometric Function4/1 -> Product5/2
  [Vc] -> Product6/1, Product5/1
  Product5/1 -> Add2/3
  Product2/1 -> Add3/1
  Trigonometric Function5/1 -> Product6/2
  Trigonometric Function3/1 -> Product4/2
  Trigonometric Function1/1 -> Product2/2
  Product4/1 -> Add3/2
  Product6/1 -> Add3/3
  Mux/1 -> Udq_m/1
  Gain/1 -> Mux/1
  Gain1/1 -> Mux/2

== system MSIP_Speed_Control_abc1a_2025a_no_VSC_no_Bspline/Motor SIncrono/Electrical Subsystem/Currents/Subsystem ==
  wrMS : Inport
  udMS : Inport  Port=2
  iqMS : Inport  Port=3
  Add4 : Sum  Inputs=-++
  Gain1 : Gain  Gain=1/Ld_MS
  Gain2 : Gain  Gain=Rs_MS
  Gain3 : Gain  Gain=np_MS*Lq_MS
  Integrator3 : Integrator  InitialCondition=0.01
  Product2 : Product
  idMS : Outport
  wires:
  Integrator3/1 -> Gain2/1, idMS/1
  Gain1/1 -> Integrator3/1
  Add4/1 -> Gain1/1
  Gain2/1 -> Add4/1
  Gain3/1 -> Add4/2
  Product2/1 -> Gain3/1
  wrMS/1 -> Product2/1
  iqMS/1 -> Product2/2
  udMS/1 -> Add4/3

== system MSIP_Speed_Control_abc1a_2025a_no_VSC_no_Bspline/Motor SIncrono/Electrical Subsystem/Currents/Subsystem1 ==
  wrMS : Inport
  uqMS : Inport  Port=2
  idMS : Inport  Port=3
  Add4 : Sum  Inputs=---+
  Gain1 : Gain  Gain=1/Lq_MS
  Gain2 : Gain  Gain=Rs_MS
  Gain3 : Gain  Gain=np_MS*Ld_MS
  Gain4 : Gain  Gain=np_MS*lambda_MS
  Integrator3 : Integrator
  Product2 : Product
  iq_Msinc : Outport
  wires:
  Product2/1 -> Gain3/1
  Gain3/1 -> Add4/2
  Gain2/1 -> Add4/1
  Add4/1 -> Gain1/1
  Gain1/1 -> Integrator3/1
  Integrator3/1 -> iq_Msinc/1, Gain2/1
  uqMS/1 -> Add4/4
  Gain4/1 -> Add4/3
  wrMS/1 -> Gain4/1, Product2/2
  idMS/1 -> Product2/1

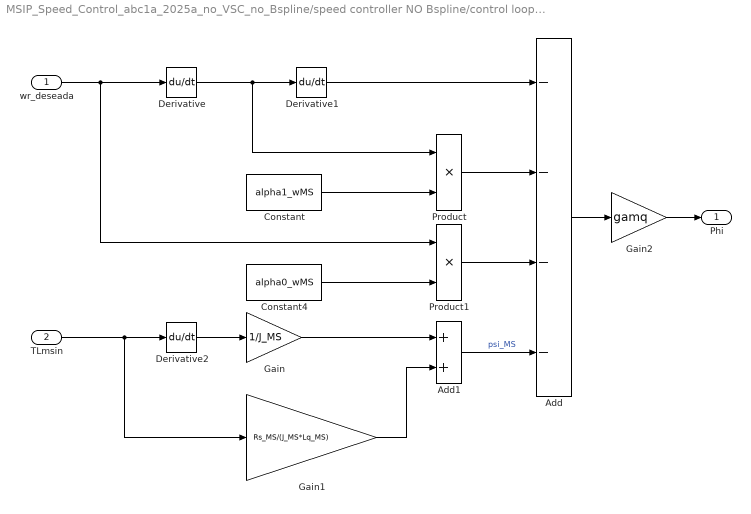
== system MSIP_Speed_Control_abc1a_2025a_no_VSC_no_Bspline/speed controller NO Bspline/control loop U_wr/Ctrl unit U1_d1/Subsystem ==
  wr_deseada : Inport
  TLmsin : Inport  Port=2
  Add : Sum  Inputs=----
  Add1 : Sum
  Constant : Constant  Value=alpha1_wMS
  Constant4 : Constant  Value=alpha0_wMS
  Derivative : Derivative
  Derivative1 : Derivative
  Derivative2 : Derivative
  Gain : Gain  Gain=1/J_MS
  Gain1 : Gain  Gain=Rs_MS/(J_MS*Lq_MS)
  Gain2 : Gain  Gain=gamq
  Product : Product
  Product1 : Product
  Phi : Outport
  wires:
  wr_deseada/1 -> Product1/1, Derivative/1
  Derivative/1 -> Product/1, Derivative1/1
  TLmsin/1 -> Derivative2/1, Gain1/1
  Derivative1/1 -> Add/1
  Product/1 -> Add/2
  Constant/1 -> Product/2
  Product1/1 -> Add/3
  Constant4/1 -> Product1/2
  Add/1 -> Gain2/1
  Gain2/1 -> Phi/1
  Add1/1 -> Add/4  "psi_MS"
  Gain/1 -> Add1/1
  Gain1/1 -> Add1/2
  Derivative2/1 -> Gain/1

== matlab function MSIP_Speed_Control_abc1a_2025a_no_VSC_no_Bspline/Subsystem/Theta_Deseada1 ==
  data: t input; ys output
function ys = theta_deseada2(t)
    
t1 = 50;   %  " initial and final instants of rest-to-rest
t2 = 60;

delt = t2-t1;
tdif = abs(t-t1) ;

% " initial and final values 
z1in = 0;
z1f  = (-100) + 1800*2*pi/60;

%z1f  = dta0;

z1dif = z1f-z1in;

tau=(tdif/delt);
tau2=tau*tau;
tau3=tau*tau2;
tau4=tau*tau3;
tau5=tau*tau4;
tau6=tau*tau5;
tau7=tau*tau6;
tau8=tau*tau7;
tau9=tau*tau8;

r1=12870;
r2=91520;
r3=288288;
r4=524160;
r5=600600;
r6=443520;
r7=205920;
r8=54912;
r9=6435;

z1st1 = z1in;
fr    = r1-r2*tau+r3*tau2-r4*tau3+r5*tau4-r6*tau5+r7*tau6-r8*tau7+r9*tau8;
z1stt = z1in+z1dif*tau8*fr;
z1st2 = z1f;


    if t<t1
         ys     = z1st1; 
    elseif t<t2
         ys     = z1stt; 
    else
         ys     = z1st2; 
    end

== matlab function MSIP_Speed_Control_abc1a_2025a_no_VSC_no_Bspline/3 Nm/TL1 ==
  data: t input; T_load output
function T_load = Tload(t)
    
t1 = 30;   %  " initial and final instants of rest-to-rest
t2 = 40;

delt = t2-t1;
tdif = abs(t-t1) ;

% " initial and final values 
z1in = 0;
z1f  = 30;

%z1f  = dta0;

z1dif = z1f-z1in;

tau=(tdif/delt);
tau2=tau*tau;
tau3=tau*tau2;
tau4=tau*tau3;
tau5=tau*tau4;
tau6=tau*tau5;
tau7=tau*tau6;
tau8=tau*tau7;
tau9=tau*tau8;

r1=12870;
r2=91520;
r3=288288;
r4=524160;
r5=600600;
r6=443520;
r7=205920;
r8=54912;
r9=6435;

z1st1 = z1in;
fr    = r1-r2*tau+r3*tau2-r4*tau3+r5*tau4-r6*tau5+r7*tau6-r8*tau7+r9*tau8;
z1stt = z1in+z1dif*tau8*fr;
z1st2 = z1f;


    if t<t1
         T_load     = z1st1; 
    elseif t<t2
         T_load     = z1stt; 
    else
         T_load     = z1st2; 
    end

== matlab function MSIP_Speed_Control_abc1a_2025a_no_VSC_no_Bspline/Subsystem/Theta_Deseada2 ==
  data: t input; ys output
function ys = theta_deseada3(t)
    
t1 = 105;   %  " initial and final instants of rest-to-rest
t2 = 110;

delt = t2-t1;
tdif = abs(t-t1) ;

% " initial and final values 
z1in = 0;
z1f  = -1600*2*pi/60;

%z1f  = dta0;

z1dif = z1f-z1in;

tau=(tdif/delt);
tau2=tau*tau;
tau3=tau*tau2;
tau4=tau*tau3;
tau5=tau*tau4;
tau6=tau*tau5;
tau7=tau*tau6;
tau8=tau*tau7;
tau9=tau*tau8;

r1=12870;
r2=91520;
r3=288288;
r4=524160;
r5=600600;
r6=443520;
r7=205920;
r8=54912;
r9=6435;

z1st1 = z1in;
fr    = r1-r2*tau+r3*tau2-r4*tau3+r5*tau4-r6*tau5+r7*tau6-r8*tau7+r9*tau8;
z1stt = z1in+z1dif*tau8*fr;
z1st2 = z1f;


    if t<t1
         ys     = z1st1; 
    elseif t<t2
         ys     = z1stt; 
    else
         ys     = z1st2; 
    end

== matlab function MSIP_Speed_Control_abc1a_2025a_no_VSC_no_Bspline/Subsystem/Theta_Deseada ==
  data: t input; ys output
function ys = theta_deseada(t)
    
t1 = 5;   %  " initial and final instants of rest-to-rest
t2 = 20;

delt = t2-t1;
tdif = abs(t-t1) ;

% " initial and final values 
z1in = 0;
z1f  = 100;


z1dif = z1f-z1in;

tau=(tdif/delt);
tau2=tau*tau;
tau3=tau*tau2;
tau4=tau*tau3;
tau5=tau*tau4;
tau6=tau*tau5;
tau7=tau*tau6;
tau8=tau*tau7;
tau9=tau*tau8;

r1=12870;
r2=91520;
r3=288288;
r4=524160;
r5=600600;
r6=443520;
r7=205920;
r8=54912;
r9=6435;

z1st1 = z1in;
fr    = r1-r2*tau+r3*tau2-r4*tau3+r5*tau4-r6*tau5+r7*tau6-r8*tau7+r9*tau8;
z1stt = z1in+z1dif*tau8*fr;
z1st2 = z1f;


    if t<t1
         ys     = z1st1; 
    elseif t<t2
         ys     = z1stt; 
    else
         ys     = z1st2; 
    end

== matlab function MSIP_Speed_Control_abc1a_2025a_no_VSC_no_Bspline/Module ==
  data: Phi_V input; angle output; Phi_I input
function angle = fcn(Phi_V,Phi_I)
   % angle = mod(Phi_V - Phi_I , 2*pi) ;
    %angle = mod(Phi_V - Phi_I , 2*pi) ;
    if (Phi_V-Phi_I<0) angle=Phi_V-Phi_I+2*pi; else angle=Phi_V-Phi_I;
end

== matlab function MSIP_Speed_Control_abc1a_2025a_no_VSC_no_Bspline/PLL1/Module ==
  data: u input; y output
function y = fcn(u)
if (and(u(1)==0,u(2)==0))
    y=1;
else
    y = sqrt(u(1)*u(1)+u(2)*u(2));
end

== matlab function MSIP_Speed_Control_abc1a_2025a_no_VSC_no_Bspline/PLL2/Module ==
  data: u input; y output
function y = fcn(u)
if (and(u(1)==0,u(2)==0))
    y=1;
else
    y = sqrt(u(1)*u(1)+u(2)*u(2));
end

== matlab function MSIP_Speed_Control_abc1a_2025a_no_VSC_no_Bspline/3 Nm/TL2 ==
  data: t input; T_load2 output
function T_load2 = Tload2(t)
    
t1 = 85;   %  " initial and final instants of rest-to-rest
t2 = 90;

delt = t2-t1;
tdif = abs(t-t1) ;

% " initial and final values 
z1in = 0;
z1f  = -25;

%z1f  = dta0;

z1dif = z1f-z1in;

tau=(tdif/delt);
tau2=tau*tau;
tau3=tau*tau2;
tau4=tau*tau3;
tau5=tau*tau4;
tau6=tau*tau5;
tau7=tau*tau6;
tau8=tau*tau7;
tau9=tau*tau8;

r1=12870;
r2=91520;
r3=288288;
r4=524160;
r5=600600;
r6=443520;
r7=205920;
r8=54912;
r9=6435;

z1st1 = z1in;
fr    = r1-r2*tau+r3*tau2-r4*tau3+r5*tau4-r6*tau5+r7*tau6-r8*tau7+r9*tau8;
z1stt = z1in+z1dif*tau8*fr;
z1st2 = z1f;


    if t<t1
         T_load2     = z1st1; 
    elseif t<t2
         T_load2     = z1stt; 
    else
         T_load2     = z1st2; 
    end

== matlab function MSIP_Speed_Control_abc1a_2025a_no_VSC_no_Bspline/3 Nm/TL3 ==
  data: t input; T_load3 output
function T_load3 = Tload3(t)
    
t1 = 125;   %  " initial and final instants of rest-to-rest
t2 = 135;

delt = t2-t1;
tdif = abs(t-t1) ;

% " initial and final values 
z1in = 0;
z1f  = 34;

%z1f  = dta0;

z1dif = z1f-z1in;

tau=(tdif/delt);
tau2=tau*tau;
tau3=tau*tau2;
tau4=tau*tau3;
tau5=tau*tau4;
tau6=tau*tau5;
tau7=tau*tau6;
tau8=tau*tau7;
tau9=tau*tau8;

r1=12870;
r2=91520;
r3=288288;
r4=524160;
r5=600600;
r6=443520;
r7=205920;
r8=54912;
r9=6435;

z1st1 = z1in;
fr    = r1-r2*tau+r3*tau2-r4*tau3+r5*tau4-r6*tau5+r7*tau6-r8*tau7+r9*tau8;
z1stt = z1in+z1dif*tau8*fr;
z1st2 = z1f;


    if t<t1
         T_load3     = z1st1; 
    elseif t<t2
         T_load3     = z1stt; 
    else
         T_load3     = z1st2; 
    end
